simulink model "Shaker_Driver_sysID2"  (Simulink 7.4)
settings: Solver=ode1  SolverMode=SingleTasking  StartTime=0.0  StopTime=inf  FixedStep=Ts  MaxStep=0.02  RelTol=1e-3  AbsTol=1e-6
PostLoadFcn:
  | global accel1 accel2 pulse;
  | Ts = 0.1
CloseFcn:
  | rtwprivate ssgencode ModelCloseRequest MC_AD
settings Model: Creator=fwornle  LastModifiedBy=fw  SimulationMode=external
settings ConfigSet: Description=rtmc9s12target_R2009b
settings DataIOCC: LimitDataPoints=off  SaveOutput=off  SaveTime=off  SignalLoggingName=sigsOut
settings OptimizationCC: BlockReduction=off  BooleanDataType=off  InitFltsAndDblsToZero=on  OptimizeModelRefInitCode=on  LifeSpan=1
settings DebuggingCC: SaveWithParameterizedLinksMsg=none  SignalResolutionControl=TryResolveAllWithWarning  SolverPrmCheckMsg=none  MultiTaskDSMMsg=warning  MultiTaskCondExecSysMsg=none  StrictBusMsg=None
settings HardwareCC: ProdBitPerInt=16  ProdEndianess=BigEndian  ProdWordSize=16  ProdHWDeviceType=Motorola HC12
settings RTWCC: SystemTargetFile=mc9s12.tlc  GenerateMakefile=off  TemplateMakefile=mc9s12.tmf  ProcessScript=mc9s12_make_rtw_hook  IncludeERTFirstTime=on
settings CodeAppCC: IgnoreCustomStorageClasses=off
settings STFCustomTargetCC: TargetFcnLib=ansi_tfl_tmw.mat  ModelReferenceCompliant=off  IncludeMdlTerminateFcn=off  ERTCustomFileBanners=on  SupportNonInlinedSFcns=off  CPPClassGenCompliant=on  SystemTargetFile=mc9s12.tlc
settings ERTTargetCC: TargetFcnLib=ansi_tfl_tmw.mat  MultiwordLength=2048  ModelReferenceCompliant=off  ParMdlRefBuildCompliant=off  CompOptLevelCompliant=off  IncludeMdlTerminateFcn=off  CombineOutputUpdateFcns=off  ERTFirstTimeCompliant=off  SupportContinuousTime=on  ModelStepFunctionPrototypeControlCompliant=off  ExtMode=on  ExtModeMexFile=ext_serial_mc9s12_comm  ExtModeMexArgs=1,2,115200  InlinedParameterPlacement=NonHierarchical  ERTCustomFileTemplate=mc9s12_file_process.tlc  GRTInterface=on  ConvertIfToSwitch=off
settings CustomProperty: DataType=RTWOptions_EnumType_C__Users_fw__SVN_rtmc9s12-target_trunk_rtmc9s12_CW_R2009b_bin_mc9s12_1mc9s12_TargetBoard  Value=Dragon12Plus
settings EnumStrPairs: String=Dragon12

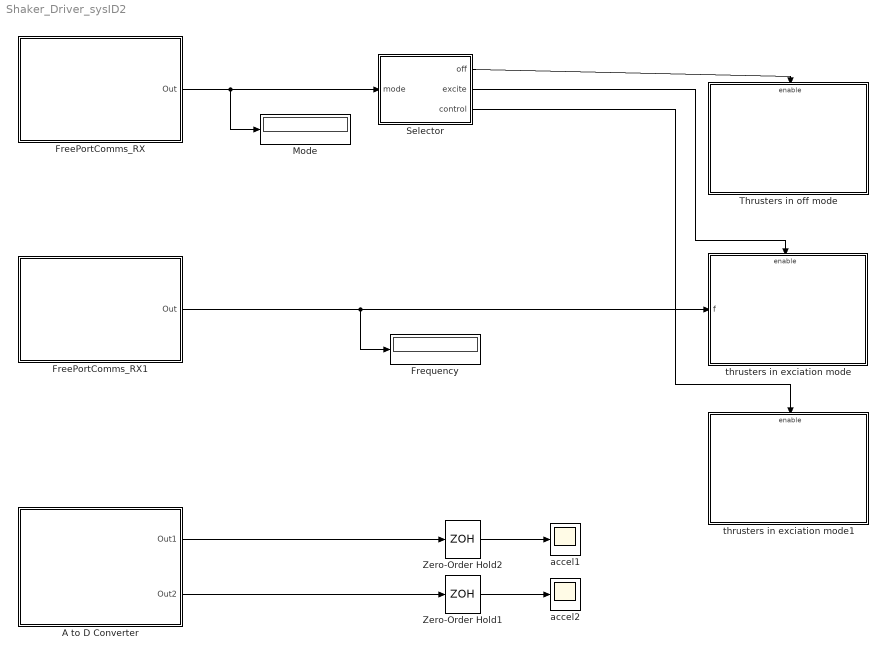
== system Shaker_Driver_sysID2 ==
  A to D Converter : Subsystem  Tag=mcTarget_adc  mask{bank=0, channels=2 3, use10bits=10 bits, normalize=max. output:  5, sampletime=Ts}
      mask prompts: bank "ADC bank"; channels "Channels ( 0 - 7 )"; use10bits "ADC resolution"; normalize "Normalization"; sampletime "Sample time"
      mask init:
      | [channelsStr, firstChannel, numChannels] = mbc_adcinput(channels);
      mask Help: web('adc_sfcn_9S12.html');
      mask StyleString: popup(0|1),edit,popup(10 bits|8 bits),popup(raw values|max. output:  1|max. output:  5),edit
      mask Display: disp(['A to D Converter\n' channelsStr])
  FreePortComms_RX : Subsystem  Tag=mcTarget_freePortCommsRX  mask{sampletime=0.1, port=SCI0, baudrate=115200, channel=0, buf_size=1, data_type=SINGLE, format=off, outformat=on}
      mask prompts: sampletime "Sample time"; port "Communication port"; channel "Channel number"; buf_size "Number of elements"; data_type "Data Type"; format "Block receives raw data"; outformat "Block output is double"
      mask init:
      | [buf_sizestr, portNamestr, baudratestr, channelstr, data_type_str, sampletime_str] = mbc_freeportrxd(sampletime, port, baudrate, channel, buf_size, data_type, format, outformat);
      mask Help: web('freePortComms_rxd.html');
      mask StyleString: edit,popup(SCI0|SCI1|COM1|COM2|COM3|COM4),popup(300|600|1200|2400|4800|9600|19200|38400|57600|115200),edit,edit,popup(SINGLE|INT8|UINT8|INT16|UINT16|INT32|UINT32|BOOLEAN),checkbox,checkbox
      mask Display: fprintf('Receive %s element(s)\nComm port: %s\nBaudrate: %s bps\nChannel: %s\nData type: %s\n Sample rate: %s', buf_sizestr, portNamestr, baudratestr, channelstr, data_type_str, sampletime_str)
  FreePortComms_RX1 : Subsystem  Tag=mcTarget_freePortCommsRX  mask{sampletime=0.1, port=SCI0, baudrate=115200, channel=1, buf_size=1, data_type=SINGLE, format=off, outformat=on}
      mask prompts: sampletime "Sample time"; port "Communication port"; channel "Channel number"; buf_size "Number of elements"; data_type "Data Type"; format "Block receives raw data"; outformat "Block output is double"
      mask init:
      | [buf_sizestr, portNamestr, baudratestr, channelstr, data_type_str, sampletime_str] = mbc_freeportrxd(sampletime, port, baudrate, channel, buf_size, data_type, format, outformat);
      mask Help: web('freePortComms_rxd.html');
      mask StyleString: edit,popup(SCI0|SCI1|COM1|COM2|COM3|COM4),popup(300|600|1200|2400|4800|9600|19200|38400|57600|115200),edit,edit,popup(SINGLE|INT8|UINT8|INT16|UINT16|INT32|UINT32|BOOLEAN),checkbox,checkbox
      mask Display: fprintf('Receive %s element(s)\nComm port: %s\nBaudrate: %s bps\nChannel: %s\nData type: %s\n Sample rate: %s', buf_sizestr, portNamestr, baudratestr, channelstr, data_type_str, sampletime_str)
  Frequency : Display
  Mode : Display
  Selector : Subsystem
  Thrusters in off mode : Subsystem
  Zero-Order Hold1 : ZeroOrderHold  SampleTime=Ts
  Zero-Order Hold2 : ZeroOrderHold  SampleTime=Ts
  accel1 : Scope
      settings: TimeRange=4  YMin=1.7  YMax=3.4  SaveName=accel1
  accel2 : Scope
      settings: TimeRange=4  YMin=-1  YMax=6  SaveName=accel2
  thrusters in exciation mode : Subsystem
  thrusters in exciation mode1 : Subsystem
  wires:
  Zero-Order Hold1/1 -> accel2/1
  A to D Converter/2(Out2) -> Zero-Order Hold1/1
  Selector/1(off) -> Thrusters in off mode/Enable
  Selector/3(control) -> thrusters in exciation mode1/Enable
  FreePortComms_RX/1(Out) -> Mode/1, Selector/1(mode)
  A to D Converter/1(Out1) -> Zero-Order Hold2/1
  Zero-Order Hold2/1 -> accel1/1
  FreePortComms_RX1/1(Out) -> thrusters in exciation mode/1(f), Frequency/1
  Selector/2(excite) -> thrusters in exciation mode/Enable

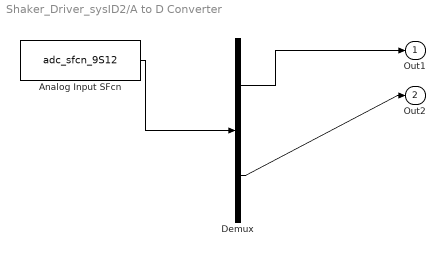
== system Shaker_Driver_sysID2/A to D Converter ==
  Analog Input SFcn : S-Function  Tag=mcTarget_adc  FunctionName=adc_sfcn_9S12  Parameters=bank-1, firstChannel, numChannels, use10bits-1, normalize, sampletime  EnableBusSupport=off
  Demux : Demux  Outputs=2
  Out1 : Outport  OutDataType=sfix(16)  OutScaling=2^0
  Out2 : Outport  Port=2
  wires:
  Analog Input SFcn/1 -> Demux/1
  Demux/1 -> Out1/1
  Demux/2 -> Out2/1

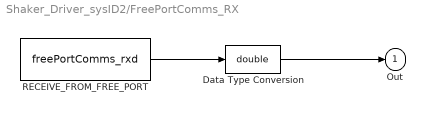
== system Shaker_Driver_sysID2/FreePortComms_RX ==
  Data Type Conversion : DataTypeConversion  OutDataTypeMode=double  OutDataType=sfix(16)  OutScaling=2^0  OutDataTypeStr=double  SaturateOnIntegerOverflow=on  RndMeth=Zero
  RECEIVE_FROM_FREE_PORT : S-Function  Tag=mcTarget_freePortCommsRX  FunctionName=freePortComms_rxd  Parameters=sampletime, channel, buf_size, data_type, port, baudrate, format  EnableBusSupport=off
  Out : Outport  OutDataType=sfix(16)  OutScaling=2^0
  wires:
  RECEIVE_FROM_FREE_PORT/1 -> Data Type Conversion/1
  Data Type Conversion/1 -> Out/1

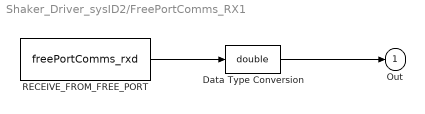
== system Shaker_Driver_sysID2/FreePortComms_RX1 ==
  Data Type Conversion : DataTypeConversion  OutDataTypeMode=double  OutDataType=sfix(16)  OutScaling=2^0  OutDataTypeStr=double  SaturateOnIntegerOverflow=on  RndMeth=Zero
  RECEIVE_FROM_FREE_PORT : S-Function  Tag=mcTarget_freePortCommsRX  FunctionName=freePortComms_rxd  Parameters=sampletime, channel, buf_size, data_type, port, baudrate, format  EnableBusSupport=off
  Out : Outport  OutDataType=sfix(16)  OutScaling=2^0
  wires:
  Data Type Conversion/1 -> Out/1
  RECEIVE_FROM_FREE_PORT/1 -> Data Type Conversion/1

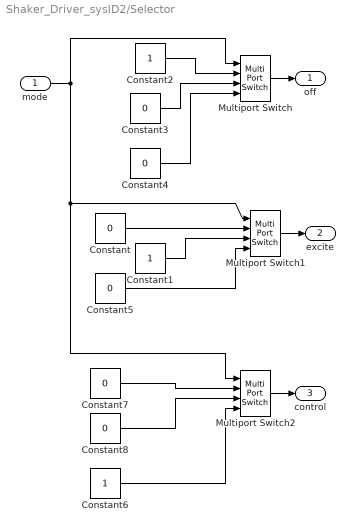
== system Shaker_Driver_sysID2/Selector ==
  mode : Inport  OutDataType=sfix(16)  OutScaling=2^0
  Constant{,3..5,7..8} (6 alike) : Constant  Value=0  OutDataType=sfix(16)  OutScaling=2^0
  Constant1 : Constant  OutDataType=sfix(16)  OutScaling=2^0
  Constant2 : Constant  OutDataType=sfix(16)  OutScaling=2^0
  Constant6 : Constant  OutDataType=sfix(16)  OutScaling=2^0
  Multiport Switch : MultiPortSwitch  SaturateOnIntegerOverflow=on
  Multiport Switch1 : MultiPortSwitch  SaturateOnIntegerOverflow=on
  Multiport Switch2 : MultiPortSwitch  SaturateOnIntegerOverflow=on
  off : Outport  OutDataType=sfix(16)  OutScaling=2^0
  excite : Outport  Port=2  OutDataType=sfix(16)  OutScaling=2^0
  control : Outport  Port=3  OutDataType=sfix(16)  OutScaling=2^0
  wires:
  Constant/1 -> Multiport Switch1/2
  Constant1/1 -> Multiport Switch1/3
  Constant4/1 -> Multiport Switch/4
  Constant3/1 -> Multiport Switch/3
  Constant2/1 -> Multiport Switch/2
  Constant5/1 -> Multiport Switch1/4
  Constant6/1 -> Multiport Switch2/4
  Constant8/1 -> Multiport Switch2/3
  Constant7/1 -> Multiport Switch2/2
  mode/1 -> Multiport Switch/1, Multiport Switch1/1, Multiport Switch2/1
  Multiport Switch/1 -> off/1
  Multiport Switch1/1 -> excite/1
  Multiport Switch2/1 -> control/1

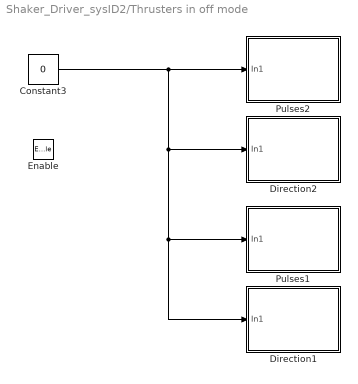
== system Shaker_Driver_sysID2/Thrusters in off mode ==
  Enable : EnablePort
  Constant3 : Constant  Value=0  OutDataType=sfix(16)  OutScaling=2^0
  Direction1 : Subsystem  Tag=mcTarget_digOut  mask{port=Port H, pin=3, sampletime=Ts, Von=0.5, Voff=0.5}
      mask prompts: port "Port (see hardware manuals for valid options)"; pin "Pin (see hardware manuals for valid options)"; sampletime "Sample time"; Von "On-threshold (Von)"; Voff "Off-threshold (Voff)"
      mask init:
      | [portstr, pinstr, pins] = mbc_digitaloutput(port, pin, sampletime, Von, Voff);
      mask Help: web('digOut_sfcn_9S12.html');
      mask StyleString: popup(Port A|Port B|Port H|Port J|Port M|Port P|Port S|Port T),edit,edit,edit,edit
      mask Display: fprintf('%s\nPins: %s', portstr, pinstr)
  Direction2 : Subsystem  Tag=mcTarget_digOut  mask{port=Port H, pin=0, sampletime=Ts, Von=0.5, Voff=0.5}
      mask prompts: port "Port (see hardware manuals for valid options)"; pin "Pin (see hardware manuals for valid options)"; sampletime "Sample time"; Von "On-threshold (Von)"; Voff "Off-threshold (Voff)"
      mask init:
      | [portstr, pinstr, pins] = mbc_digitaloutput(port, pin, sampletime, Von, Voff);
      mask Help: web('digOut_sfcn_9S12.html');
      mask StyleString: popup(Port A|Port B|Port H|Port J|Port M|Port P|Port S|Port T),edit,edit,edit,edit
      mask Display: fprintf('%s\nPins: %s', portstr, pinstr)
  Pulses1 : Subsystem  Tag=mcTarget_digOut  mask{port=Port H, pin=2, sampletime=Ts, Von=0.5, Voff=0.5}
      mask prompts: port "Port (see hardware manuals for valid options)"; pin "Pin (see hardware manuals for valid options)"; sampletime "Sample time"; Von "On-threshold (Von)"; Voff "Off-threshold (Voff)"
      mask init:
      | [portstr, pinstr, pins] = mbc_digitaloutput(port, pin, sampletime, Von, Voff);
      mask Help: web('digOut_sfcn_9S12.html');
      mask StyleString: popup(Port A|Port B|Port H|Port J|Port M|Port P|Port S|Port T),edit,edit,edit,edit
      mask Display: fprintf('%s\nPins: %s', portstr, pinstr)
  Pulses2 : Subsystem  Tag=mcTarget_digOut  mask{port=Port H, pin=1, sampletime=Ts, Von=0.5, Voff=0.5}
      mask prompts: port "Port (see hardware manuals for valid options)"; pin "Pin (see hardware manuals for valid options)"; sampletime "Sample time"; Von "On-threshold (Von)"; Voff "Off-threshold (Voff)"
      mask init:
      | [portstr, pinstr, pins] = mbc_digitaloutput(port, pin, sampletime, Von, Voff);
      mask Help: web('digOut_sfcn_9S12.html');
      mask StyleString: popup(Port A|Port B|Port H|Port J|Port M|Port P|Port S|Port T),edit,edit,edit,edit
      mask Display: fprintf('%s\nPins: %s', portstr, pinstr)
  wires:
  Constant3/1 -> Pulses1/1(In1), Direction1/1(In1), Direction2/1(In1), Pulses2/1(In1)

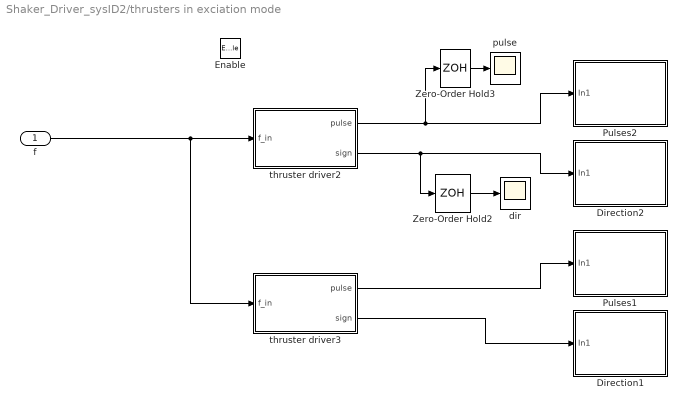
== system Shaker_Driver_sysID2/thrusters in exciation mode ==
  f : Inport  OutDataType=sfix(16)  OutScaling=2^0
  Enable : EnablePort
  Direction1 : Subsystem  Tag=mcTarget_digOut  mask{port=Port H, pin=3, sampletime=Ts, Von=0.5, Voff=0.5}
      mask prompts: port "Port (see hardware manuals for valid options)"; pin "Pin (see hardware manuals for valid options)"; sampletime "Sample time"; Von "On-threshold (Von)"; Voff "Off-threshold (Voff)"
      mask init:
      | [portstr, pinstr, pins] = mbc_digitaloutput(port, pin, sampletime, Von, Voff);
      mask Help: web('digOut_sfcn_9S12.html');
      mask StyleString: popup(Port A|Port B|Port H|Port J|Port M|Port P|Port S|Port T),edit,edit,edit,edit
      mask Display: fprintf('%s\nPins: %s', portstr, pinstr)
  Direction2 : Subsystem  Tag=mcTarget_digOut  mask{port=Port H, pin=0, sampletime=Ts, Von=0.5, Voff=0.5}
      mask prompts: port "Port (see hardware manuals for valid options)"; pin "Pin (see hardware manuals for valid options)"; sampletime "Sample time"; Von "On-threshold (Von)"; Voff "Off-threshold (Voff)"
      mask init:
      | [portstr, pinstr, pins] = mbc_digitaloutput(port, pin, sampletime, Von, Voff);
      mask Help: web('digOut_sfcn_9S12.html');
      mask StyleString: popup(Port A|Port B|Port H|Port J|Port M|Port P|Port S|Port T),edit,edit,edit,edit
      mask Display: fprintf('%s\nPins: %s', portstr, pinstr)
  Pulses1 : Subsystem  Tag=mcTarget_digOut  mask{port=Port H, pin=2, sampletime=Ts, Von=0.5, Voff=0.5}
      mask prompts: port "Port (see hardware manuals for valid options)"; pin "Pin (see hardware manuals for valid options)"; sampletime "Sample time"; Von "On-threshold (Von)"; Voff "Off-threshold (Voff)"
      mask init:
      | [portstr, pinstr, pins] = mbc_digitaloutput(port, pin, sampletime, Von, Voff);
      mask Help: web('digOut_sfcn_9S12.html');
      mask StyleString: popup(Port A|Port B|Port H|Port J|Port M|Port P|Port S|Port T),edit,edit,edit,edit
      mask Display: fprintf('%s\nPins: %s', portstr, pinstr)
  Pulses2 : Subsystem  Tag=mcTarget_digOut  mask{port=Port H, pin=1, sampletime=Ts, Von=0.5, Voff=0.5}
      mask prompts: port "Port (see hardware manuals for valid options)"; pin "Pin (see hardware manuals for valid options)"; sampletime "Sample time"; Von "On-threshold (Von)"; Voff "Off-threshold (Voff)"
      mask init:
      | [portstr, pinstr, pins] = mbc_digitaloutput(port, pin, sampletime, Von, Voff);
      mask Help: web('digOut_sfcn_9S12.html');
      mask StyleString: popup(Port A|Port B|Port H|Port J|Port M|Port P|Port S|Port T),edit,edit,edit,edit
      mask Display: fprintf('%s\nPins: %s', portstr, pinstr)
  Zero-Order Hold2 : ZeroOrderHold  SampleTime=Ts
  Zero-Order Hold3 : ZeroOrderHold  SampleTime=Ts
  dir : Scope
      settings: TimeRange=4  YMin=-1  YMax=2  SaveName=direction
  pulse : Scope
      settings: TimeRange=4  YMin=-1  YMax=2  SaveName=pulse
  thruster driver2 : Subsystem
  thruster driver3 : Subsystem
  wires:
  Zero-Order Hold3/1 -> pulse/1
  Zero-Order Hold2/1 -> dir/1
  thruster driver3/2(sign) -> Direction1/1(In1)
  thruster driver3/1(pulse) -> Pulses1/1(In1)
  thruster driver2/1(pulse) -> Zero-Order Hold3/1, Pulses2/1(In1)
  thruster driver2/2(sign) -> Zero-Order Hold2/1, Direction2/1(In1)
  f/1 -> thruster driver2/1(f_in), thruster driver3/1(f_in)

== system Shaker_Driver_sysID2/thrusters in exciation mode1 ==
  Enable : EnablePort

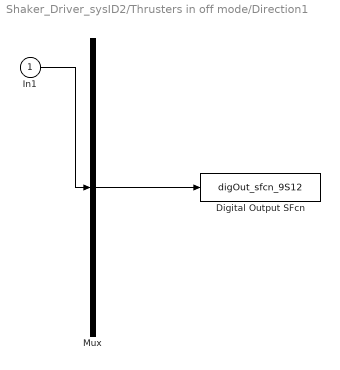
== system Shaker_Driver_sysID2/Thrusters in off mode/Direction1 ==
  In1 : Inport  OutDataType=sfix(16)  OutScaling=2^0
  Digital Output SFcn : S-Function  Tag=mcTarget_digOut  FunctionName=digOut_sfcn_9S12  Parameters=sampletime, port, pins, Von, Voff  EnableBusSupport=off
  Mux : Mux  Inputs=1
  wires:
  Mux/1 -> Digital Output SFcn/1
  In1/1 -> Mux/1

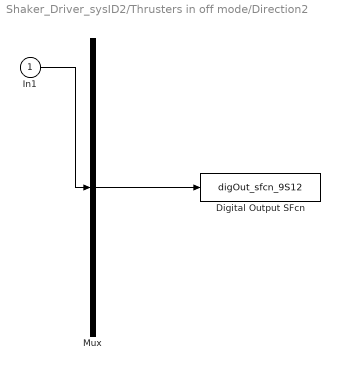
== system Shaker_Driver_sysID2/Thrusters in off mode/Direction2 ==
  In1 : Inport  OutDataType=sfix(16)  OutScaling=2^0
  Digital Output SFcn : S-Function  Tag=mcTarget_digOut  FunctionName=digOut_sfcn_9S12  Parameters=sampletime, port, pins, Von, Voff  EnableBusSupport=off
  Mux : Mux  Inputs=1
  wires:
  In1/1 -> Mux/1
  Mux/1 -> Digital Output SFcn/1

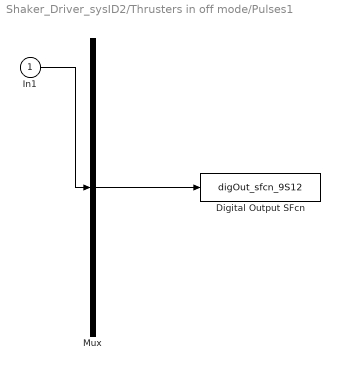
== system Shaker_Driver_sysID2/Thrusters in off mode/Pulses1 ==
  In1 : Inport  OutDataType=sfix(16)  OutScaling=2^0
  Digital Output SFcn : S-Function  Tag=mcTarget_digOut  FunctionName=digOut_sfcn_9S12  Parameters=sampletime, port, pins, Von, Voff  EnableBusSupport=off
  Mux : Mux  Inputs=1
  wires:
  Mux/1 -> Digital Output SFcn/1
  In1/1 -> Mux/1

== system Shaker_Driver_sysID2/Thrusters in off mode/Pulses2 ==
  In1 : Inport  OutDataType=sfix(16)  OutScaling=2^0
  Digital Output SFcn : S-Function  Tag=mcTarget_digOut  FunctionName=digOut_sfcn_9S12  Parameters=sampletime, port, pins, Von, Voff  EnableBusSupport=off
  Mux : Mux  Inputs=1
  wires:
  In1/1 -> Mux/1
  Mux/1 -> Digital Output SFcn/1

== system Shaker_Driver_sysID2/thrusters in exciation mode/Direction1 ==
  In1 : Inport  OutDataType=sfix(16)  OutScaling=2^0
  Digital Output SFcn : S-Function  Tag=mcTarget_digOut  FunctionName=digOut_sfcn_9S12  Parameters=sampletime, port, pins, Von, Voff  EnableBusSupport=off
  Mux : Mux  Inputs=1
  wires:
  Mux/1 -> Digital Output SFcn/1
  In1/1 -> Mux/1

== system Shaker_Driver_sysID2/thrusters in exciation mode/Direction2 ==
  In1 : Inport  OutDataType=sfix(16)  OutScaling=2^0
  Digital Output SFcn : S-Function  Tag=mcTarget_digOut  FunctionName=digOut_sfcn_9S12  Parameters=sampletime, port, pins, Von, Voff  EnableBusSupport=off
  Mux : Mux  Inputs=1
  wires:
  In1/1 -> Mux/1
  Mux/1 -> Digital Output SFcn/1

== system Shaker_Driver_sysID2/thrusters in exciation mode/Pulses1 ==
  In1 : Inport  OutDataType=sfix(16)  OutScaling=2^0
  Digital Output SFcn : S-Function  Tag=mcTarget_digOut  FunctionName=digOut_sfcn_9S12  Parameters=sampletime, port, pins, Von, Voff  EnableBusSupport=off
  Mux : Mux  Inputs=1
  wires:
  Mux/1 -> Digital Output SFcn/1
  In1/1 -> Mux/1

== system Shaker_Driver_sysID2/thrusters in exciation mode/Pulses2 ==
  In1 : Inport  OutDataType=sfix(16)  OutScaling=2^0
  Digital Output SFcn : S-Function  Tag=mcTarget_digOut  FunctionName=digOut_sfcn_9S12  Parameters=sampletime, port, pins, Von, Voff  EnableBusSupport=off
  Mux : Mux  Inputs=1
  wires:
  In1/1 -> Mux/1
  Mux/1 -> Digital Output SFcn/1

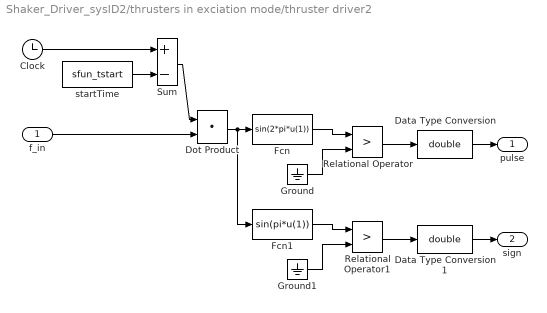
== system Shaker_Driver_sysID2/thrusters in exciation mode/thruster driver2 ==
  f_in : Inport  OutDataType=sfix(16)  OutScaling=2^0
  Clock : Clock
      settings: Decimation=10
  Data Type Conversion : DataTypeConversion  OutDataTypeMode=double  OutDataType=sfix(16)  OutScaling=2^0  OutDataTypeStr=double  SaturateOnIntegerOverflow=on  RndMeth=Zero
  Data Type Conversion1 : DataTypeConversion  OutDataTypeMode=double  OutDataType=sfix(16)  OutScaling=2^0  OutDataTypeStr=double  SaturateOnIntegerOverflow=on  RndMeth=Zero
  Dot Product : DotProduct  OutDataType=sfix(16)  OutScaling=2^-10  InputSameDT=on  OutDataTypeStr=Inherit: Inherit via internal rule
  Fcn : Fcn  Expr=sin(2*pi*u(1))
  Fcn1 : Fcn  Expr=sin(pi*u(1))
  Ground : Ground
  Ground1 : Ground
  Relational Operator : RelationalOperator  Operator=>  InputSameDT=on
  Relational Operator1 : RelationalOperator  Operator=>  InputSameDT=on
  Sum : Sum  Inputs=+-  OutDataType=sfix(16)  OutScaling=2^0  SaturateOnIntegerOverflow=on  InputSameDT=on  OutDataTypeStr=Inherit: Same as first input
  startTime : S-Function  FunctionName=sfun_tstart  EnableBusSupport=off
  pulse : Outport  OutDataType=sfix(16)  OutScaling=2^0
  sign : Outport  Port=2  OutDataType=sfix(16)  OutScaling=2^0
  wires:
  Data Type Conversion1/1 -> sign/1
  Relational Operator1/1 -> Data Type Conversion1/1
  Ground1/1 -> Relational Operator1/2
  Fcn1/1 -> Relational Operator1/1
  Data Type Conversion/1 -> pulse/1
  f_in/1 -> Dot Product/2
  Sum/1 -> Dot Product/1
  Relational Operator/1 -> Data Type Conversion/1
  Ground/1 -> Relational Operator/2
  Fcn/1 -> Relational Operator/1
  Dot Product/1 -> Fcn1/1, Fcn/1
  Clock/1 -> Sum/1
  startTime/1 -> Sum/2

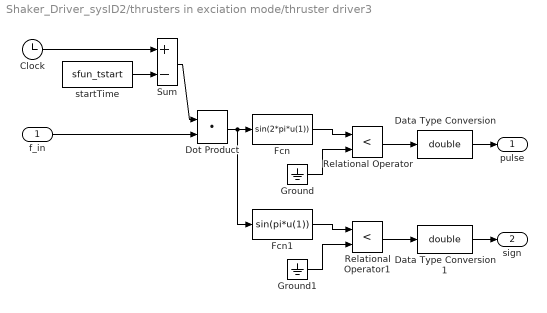
== system Shaker_Driver_sysID2/thrusters in exciation mode/thruster driver3 ==
  f_in : Inport  OutDataType=sfix(16)  OutScaling=2^0
  Clock : Clock
      settings: Decimation=10
  Data Type Conversion : DataTypeConversion  OutDataTypeMode=double  OutDataType=sfix(16)  OutScaling=2^0  OutDataTypeStr=double  SaturateOnIntegerOverflow=on  RndMeth=Zero
  Data Type Conversion1 : DataTypeConversion  OutDataTypeMode=double  OutDataType=sfix(16)  OutScaling=2^0  OutDataTypeStr=double  SaturateOnIntegerOverflow=on  RndMeth=Zero
  Dot Product : DotProduct  OutDataType=sfix(16)  OutScaling=2^-10  InputSameDT=on  OutDataTypeStr=Inherit: Inherit via internal rule
  Fcn : Fcn  Expr=sin(2*pi*u(1))
  Fcn1 : Fcn  Expr=sin(pi*u(1))
  Ground : Ground
  Ground1 : Ground
  Relational Operator : RelationalOperator  Operator=<  InputSameDT=on
  Relational Operator1 : RelationalOperator  Operator=<  InputSameDT=on
  Sum : Sum  Inputs=+-  OutDataType=sfix(16)  OutScaling=2^0  SaturateOnIntegerOverflow=on  InputSameDT=on  OutDataTypeStr=Inherit: Same as first input
  startTime : S-Function  FunctionName=sfun_tstart  EnableBusSupport=off
  pulse : Outport  OutDataType=sfix(16)  OutScaling=2^0
  sign : Outport  Port=2  OutDataType=sfix(16)  OutScaling=2^0
  wires:
  startTime/1 -> Sum/2
  Clock/1 -> Sum/1
  Dot Product/1 -> Fcn/1, Fcn1/1
  Fcn/1 -> Relational Operator/1
  Ground/1 -> Relational Operator/2
  Relational Operator/1 -> Data Type Conversion/1
  Sum/1 -> Dot Product/1
  f_in/1 -> Dot Product/2
  Data Type Conversion/1 -> pulse/1
  Fcn1/1 -> Relational Operator1/1
  Ground1/1 -> Relational Operator1/2
  Relational Operator1/1 -> Data Type Conversion1/1
  Data Type Conversion1/1 -> sign/1
